simulink model "Lab3_sim"  (R2020a)
settings: Solver=VariableStepAuto  StartTime=0.0  StopTime=10.0  RelTol=1e-3
settings Model: Creator=adamj  LastModifiedBy=adamj

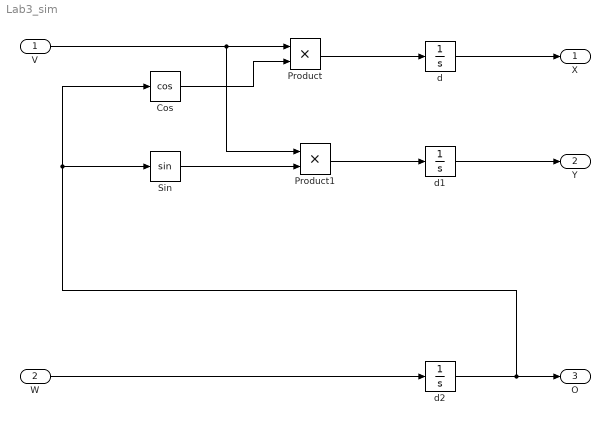
== system Lab3_sim ==
  V : Inport
  W : Inport  Port=2
  Cos : Trigonometry  Operator=cos
  Product : Product
  Product1 : Product
  Sin : Trigonometry
  d : Integrator  InitialCondition=1/4
  d1 : Integrator  InitialCondition=1/4
  d2 : Integrator  InitialCondition=1/4
  X : Outport
  Y : Outport  Port=2
  O : Outport  Port=3
  wires:
  d/1 -> X/1
  d1/1 -> Y/1
  d2/1 -> Sin/1, Cos/1, O/1
  W/1 -> d2/1
  Cos/1 -> Product/2
  V/1 -> Product1/1, Product/1
  Sin/1 -> Product1/2
  Product1/1 -> d1/1
  Product/1 -> d/1
